simulink model "CycleSend_2018a"  (R2018a)
settings: Solver=VariableStepAuto  StartTime=0.0  StopTime=10.0  RelTol=1e-3
settings Model: Creator=apple  LastModifiedBy=apple
settings DataIOCC: ReturnWorkspaceOutputs=on
settings SFSimCC: SimUseLocalCustomCode=on
settings RTWCC: RTWUseLocalCustomCode=on

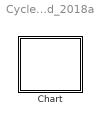
== system CycleSend_2018a ==
  Chart : Stateflow chart  TreatAsAtomicUnit=on

== stateflow chart CycleSend_2018a/Chart ==
  state On
    en:fprintf("Entry On");
    du:fprintf("During On");
    ex:fprintf("Exit On");
  state Off
    en:fprintf("Entry Off");
    du:fprintf("During Off");
    ex:fprintf("Exit Off");
  (default) -> On
  On -> Off : E_one{send(E_one);}
  Off -> On : E_one
  events: E_one local FUNCTION_CALL_EVENT
